simulink model "FTD_test"  (R2023a)
settings: Solver=FixedStepAuto  StartTime=0.0  StopTime=150  FixedStep=0.001  RelTol=1e-3
libraries: simulink x2
settings Model: Creator=邓宇飞  LastModifiedBy=邓宇飞

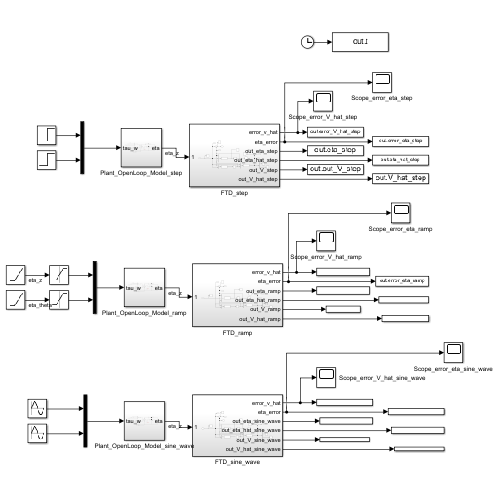
[thumbnail: Simulink's stored preview of the top-level diagram]
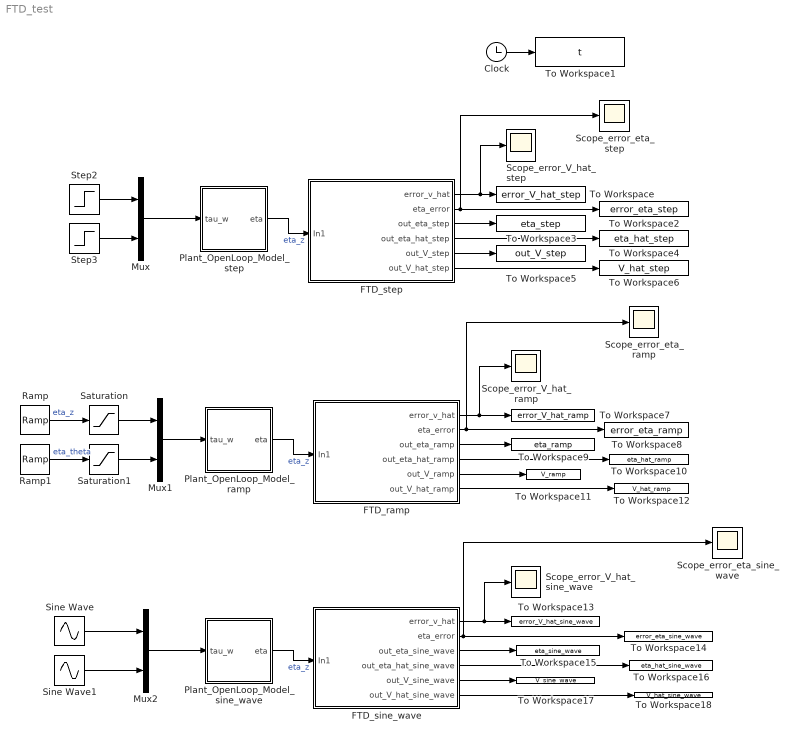
== system FTD_test ==
  Clock : Clock
  FTD_ramp : Subsystem
  FTD_sine_wave : Subsystem
  FTD_step : Subsystem
  Mux : Mux  Inputs=2
  Mux1 : Mux  Inputs=2
  Mux2 : Mux  Inputs=2
  Plant_OpenLoop_Model_ramp : Subsystem
  Plant_OpenLoop_Model_sine_wave : Subsystem
  Plant_OpenLoop_Model_step : Subsystem
  Ramp : simulink/Sources/Ramp  slope=1  start=1  InitialOutput=0
  Ramp1 : simulink/Sources/Ramp  slope=1  start=1  InitialOutput=0
  Saturation : Saturate  UpperLimit=10  LowerLimit=0
  Saturation1 : Saturate  UpperLimit=10  LowerLimit=0
  Scope_error_V_hat_ramp : Scope
  Scope_error_V_hat_sine_wave : Scope
  Scope_error_V_hat_step : Scope
  Scope_error_eta_ramp : Scope
  Scope_error_eta_sine_wave : Scope
  Scope_error_eta_step : Scope
  Sine Wave : Sin  Frequency=0.5*pi  Phase=0.5*pi  SampleTime=0
  Sine Wave1 : Sin  Frequency=0.5*pi  Phase=0.5*pi  SampleTime=0
  Step2 : Step  Time=0  SampleTime=0
  Step3 : Step  Time=0  SampleTime=0
  To Workspace : ToWorkspace  VariableName=error_V_hat_step  SaveFormat=Timeseries  SampleTime=-1
  To Workspace1 : ToWorkspace  VariableName=t  SaveFormat=Timeseries  SampleTime=-1
  To Workspace10 : ToWorkspace  VariableName=eta_hat_ramp  SaveFormat=Timeseries  SampleTime=-1
  To Workspace11 : ToWorkspace  VariableName=V_ramp  SaveFormat=Timeseries  SampleTime=-1
  To Workspace12 : ToWorkspace  VariableName=V_hat_ramp  SaveFormat=Timeseries  SampleTime=-1
  To Workspace13 : ToWorkspace  VariableName=error_V_hat_sine_wave  SaveFormat=Timeseries  SampleTime=-1
  To Workspace14 : ToWorkspace  VariableName=error_eta_sine_wave  SaveFormat=Timeseries  SampleTime=-1
  To Workspace15 : ToWorkspace  VariableName=eta_sine_wave  SaveFormat=Timeseries  SampleTime=-1
  To Workspace16 : ToWorkspace  VariableName=eta_hat_sine_wave  SaveFormat=Timeseries  SampleTime=-1
  To Workspace17 : ToWorkspace  VariableName=V_sine_wave  SaveFormat=Timeseries  SampleTime=-1
  To Workspace18 : ToWorkspace  VariableName=V_hat_sine_wave  SaveFormat=Timeseries  SampleTime=-1
  To Workspace2 : ToWorkspace  VariableName=error_eta_step  SaveFormat=Timeseries  SampleTime=-1
  To Workspace3 : ToWorkspace  VariableName=eta_step  SaveFormat=Timeseries  SampleTime=-1
  To Workspace4 : ToWorkspace  VariableName=eta_hat_step  SaveFormat=Timeseries  SampleTime=-1
  To Workspace5 : ToWorkspace  VariableName=out_V_step  SaveFormat=Timeseries  SampleTime=-1
  To Workspace6 : ToWorkspace  VariableName=V_hat_step  SaveFormat=Timeseries  SampleTime=-1
  To Workspace7 : ToWorkspace  VariableName=error_V_hat_ramp  SaveFormat=Timeseries  SampleTime=-1
  To Workspace8 : ToWorkspace  VariableName=error_eta_ramp  SaveFormat=Timeseries  SampleTime=-1
  To Workspace9 : ToWorkspace  VariableName=eta_ramp  SaveFormat=Timeseries  SampleTime=-1
  wires:
  Plant_OpenLoop_Model_step/1(eta) -> FTD_step/1(In1)  "eta_z"
  FTD_step/1(error_v_hat) -> Scope_error_V_hat_step/1, To Workspace/1
  FTD_step/2(eta_error) -> To Workspace2/1, Scope_error_eta_step/1
  FTD_ramp/2(eta_error) -> To Workspace8/1, Scope_error_eta_ramp/1
  FTD_ramp/1(error_v_hat) -> To Workspace7/1, Scope_error_V_hat_ramp/1
  Plant_OpenLoop_Model_ramp/1(eta) -> FTD_ramp/1(In1)  "eta_z"
  FTD_sine_wave/2(eta_error) -> To Workspace14/1, Scope_error_eta_sine_wave/1
  FTD_sine_wave/1(error_v_hat) -> To Workspace13/1, Scope_error_V_hat_sine_wave/1
  Plant_OpenLoop_Model_sine_wave/1(eta) -> FTD_sine_wave/1(In1)  "eta_z"
  Mux/1 -> Plant_OpenLoop_Model_step/1(tau_w)
  Step2/1 -> Mux/1
  Step3/1 -> Mux/2
  Mux1/1 -> Plant_OpenLoop_Model_ramp/1(tau_w)
  Saturation1/1 -> Mux1/2
  Saturation/1 -> Mux1/1
  Ramp/1 -> Saturation/1  "eta_z"
  Ramp1/1 -> Saturation1/1  "eta_theta"
  Mux2/1 -> Plant_OpenLoop_Model_sine_wave/1(tau_w)
  Sine Wave/1 -> Mux2/1
  Sine Wave1/1 -> Mux2/2
  FTD_step/3(out_eta_step) -> To Workspace3/1
  FTD_step/4(out_eta_hat_step) -> To Workspace4/1
  FTD_step/6(out_V_hat_step) -> To Workspace6/1
  FTD_ramp/3(out_eta_ramp) -> To Workspace9/1
  FTD_ramp/4(out_eta_hat_ramp) -> To Workspace10/1
  FTD_ramp/5(out_V_ramp) -> To Workspace11/1
  FTD_ramp/6(out_V_hat_ramp) -> To Workspace12/1
  FTD_sine_wave/3(out_eta_sine_wave) -> To Workspace15/1
  FTD_sine_wave/4(out_eta_hat_sine_wave) -> To Workspace16/1
  FTD_sine_wave/5(out_V_sine_wave) -> To Workspace17/1
  FTD_sine_wave/6(out_V_hat_sine_wave) -> To Workspace18/1
  Clock/1 -> To Workspace1/1
  FTD_step/5(out_V_step) -> To Workspace5/1

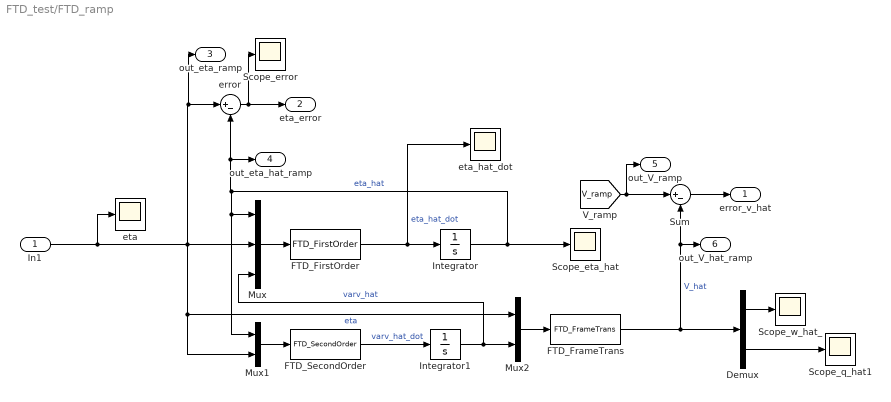
== system FTD_test/FTD_ramp ==
  In1 : Inport
  Demux : Demux  Outputs=2
  FTD_FirstOrder : MATLABFcn  MATLABFcn=FTD_FirstOrder  OutputDimensions=2  OutputSignalType=real
  FTD_FrameTrans : MATLABFcn  MATLABFcn=FTD_FrameTrans  OutputDimensions=2  OutputSignalType=real
  FTD_SecondOrder : MATLABFcn  MATLABFcn=FTD_SecondOrder  OutputDimensions=2  OutputSignalType=real
  Integrator : Integrator
  Integrator1 : Integrator
  Mux : Mux  Inputs=3
  Mux1 : Mux  Inputs=2
  Mux2 : Mux  Inputs=2
  Scope_error : Scope
  Scope_eta_hat : Scope
  Scope_q_hat1 : Scope
  Scope_w_hat_ : Scope
  Sum : Sum  Inputs=|+-
  error : Sum  Inputs=|+-
  eta : Scope
  eta_hat_dot : Scope
  error_v_hat : Outport
  eta_error : Outport  Port=2
  out_eta_ramp : Outport  Port=3
  out_eta_hat_ramp : Outport  Port=4
  out_V_ramp : Outport  Port=5
  out_V_hat_ramp : Outport  Port=6
  wires:
  In1/1 -> eta/1, out_eta_ramp/1, error/1, Mux2/1, Mux1/2, Mux/2  "eta"
  Mux/1 -> FTD_FirstOrder/1
  Integrator/1 -> Scope_eta_hat/1, out_eta_hat_ramp/1, error/2, Mux1/1, Mux/1  "eta_hat"
  FTD_FrameTrans/1 -> Demux/1, out_V_hat_ramp/1, Sum/2  "V_hat"
  FTD_FirstOrder/1 -> Integrator/1, eta_hat_dot/1  "eta_hat_dot"
  error/1 -> eta_error/1, Scope_error/1
  Demux/1 -> Scope_w_hat_/1
  FTD_SecondOrder/1 -> Integrator1/1  "varv_hat_dot"
  Integrator1/1 -> Mux/3, Mux2/2  "varv_hat"
  Mux1/1 -> FTD_SecondOrder/1
  Mux2/1 -> FTD_FrameTrans/1
  Demux/2 -> Scope_q_hat1/1
  [V_ramp] -> out_V_ramp/1, Sum/1
  Sum/1 -> error_v_hat/1

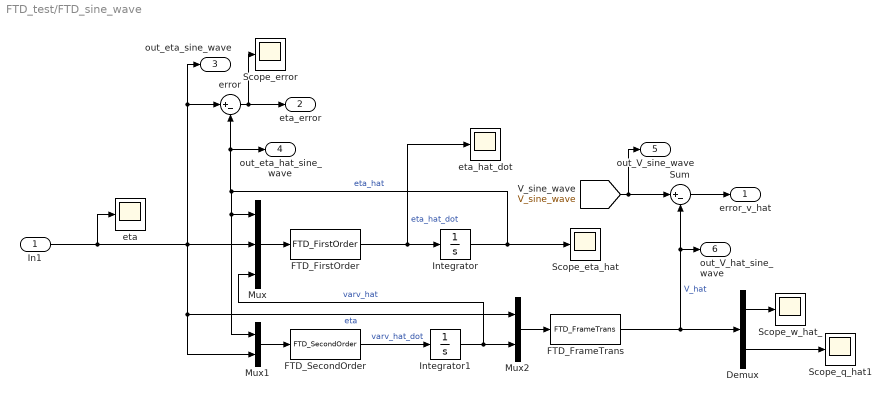
== system FTD_test/FTD_sine_wave ==
  In1 : Inport
  Demux : Demux  Outputs=2
  FTD_FirstOrder : MATLABFcn  MATLABFcn=FTD_FirstOrder  OutputDimensions=2  OutputSignalType=real
  FTD_FrameTrans : MATLABFcn  MATLABFcn=FTD_FrameTrans  OutputDimensions=2  OutputSignalType=real
  FTD_SecondOrder : MATLABFcn  MATLABFcn=FTD_SecondOrder  OutputDimensions=2  OutputSignalType=real
  Integrator : Integrator
  Integrator1 : Integrator
  Mux : Mux  Inputs=3
  Mux1 : Mux  Inputs=2
  Mux2 : Mux  Inputs=2
  Scope_error : Scope
  Scope_eta_hat : Scope
  Scope_q_hat1 : Scope
  Scope_w_hat_ : Scope
  Sum : Sum  Inputs=|+-
  error : Sum  Inputs=|+-
  eta : Scope
  eta_hat_dot : Scope
  error_v_hat : Outport
  eta_error : Outport  Port=2
  out_eta_sine_wave : Outport  Port=3
  out_eta_hat_sine_wave : Outport  Port=4
  out_V_sine_wave : Outport  Port=5
  out_V_hat_sine_wave : Outport  Port=6
  wires:
  In1/1 -> eta/1, out_eta_sine_wave/1, error/1, Mux2/1, Mux1/2, Mux/2  "eta"
  Mux/1 -> FTD_FirstOrder/1
  Integrator/1 -> Scope_eta_hat/1, out_eta_hat_sine_wave/1, error/2, Mux1/1, Mux/1  "eta_hat"
  FTD_FrameTrans/1 -> Demux/1, out_V_hat_sine_wave/1, Sum/2  "V_hat"
  FTD_FirstOrder/1 -> Integrator/1, eta_hat_dot/1  "eta_hat_dot"
  error/1 -> eta_error/1, Scope_error/1
  Demux/1 -> Scope_w_hat_/1
  FTD_SecondOrder/1 -> Integrator1/1  "varv_hat_dot"
  Integrator1/1 -> Mux/3, Mux2/2  "varv_hat"
  Mux1/1 -> FTD_SecondOrder/1
  Mux2/1 -> FTD_FrameTrans/1
  Demux/2 -> Scope_q_hat1/1
  [V_sine_wave] -> out_V_sine_wave/1, Sum/1
  Sum/1 -> error_v_hat/1

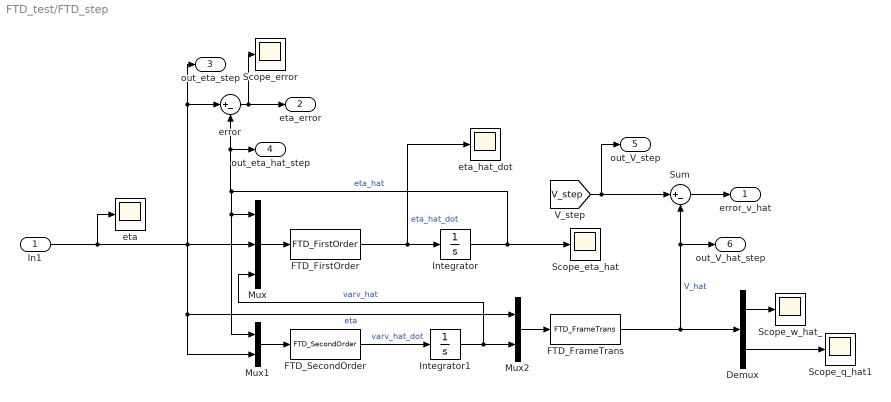
== system FTD_test/FTD_step ==
  In1 : Inport
  Demux : Demux  Outputs=2
  FTD_FirstOrder : MATLABFcn  MATLABFcn=FTD_FirstOrder  OutputDimensions=2  OutputSignalType=real
  FTD_FrameTrans : MATLABFcn  MATLABFcn=FTD_FrameTrans  OutputDimensions=2  OutputSignalType=real
  FTD_SecondOrder : MATLABFcn  MATLABFcn=FTD_SecondOrder  OutputDimensions=2  OutputSignalType=real
  Integrator : Integrator
  Integrator1 : Integrator
  Mux : Mux  Inputs=3
  Mux1 : Mux  Inputs=2
  Mux2 : Mux  Inputs=2
  Scope_error : Scope
  Scope_eta_hat : Scope
  Scope_q_hat1 : Scope
  Scope_w_hat_ : Scope
  Sum : Sum  Inputs=|+-
  error : Sum  Inputs=|+-
  eta : Scope
  eta_hat_dot : Scope
  error_v_hat : Outport
  eta_error : Outport  Port=2
  out_eta_step : Outport  Port=3
  out_eta_hat_step : Outport  Port=4
  out_V_step : Outport  Port=5
  out_V_hat_step : Outport  Port=6
  wires:
  In1/1 -> eta/1, error/1, out_eta_step/1, Mux2/1, Mux1/2, Mux/2  "eta"
  Mux/1 -> FTD_FirstOrder/1
  Integrator/1 -> Scope_eta_hat/1, out_eta_hat_step/1, error/2, Mux1/1, Mux/1  "eta_hat"
  FTD_FrameTrans/1 -> Demux/1, out_V_hat_step/1, Sum/2  "V_hat"
  FTD_FirstOrder/1 -> Integrator/1, eta_hat_dot/1  "eta_hat_dot"
  error/1 -> eta_error/1, Scope_error/1
  Demux/1 -> Scope_w_hat_/1
  FTD_SecondOrder/1 -> Integrator1/1  "varv_hat_dot"
  Integrator1/1 -> Mux/3, Mux2/2  "varv_hat"
  Mux1/1 -> FTD_SecondOrder/1
  Mux2/1 -> FTD_FrameTrans/1
  Demux/2 -> Scope_q_hat1/1
  [V_step] -> Sum/1, out_V_step/1
  Sum/1 -> error_v_hat/1

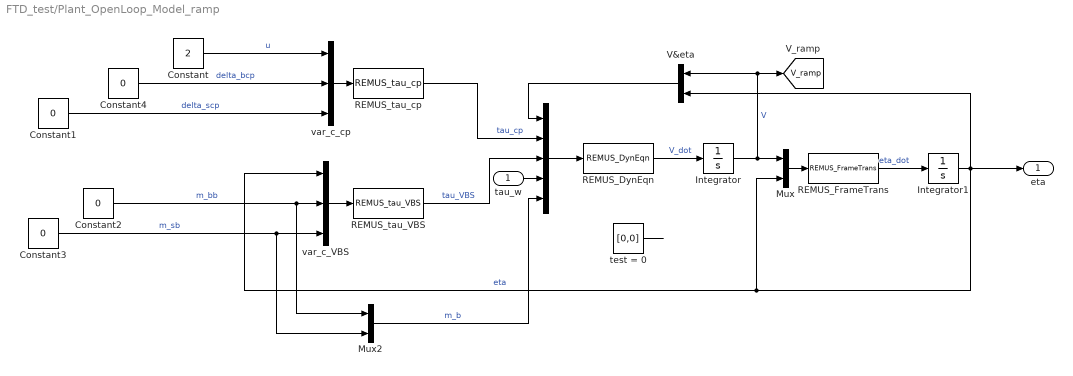
== system FTD_test/Plant_OpenLoop_Model_ramp ==
  tau_w : Inport
  " " : Mux  Inputs=5
  Constant : Constant  Value=2  OutDataTypeStr=Inherit: Inherit via back propagation
  Constant{1..4} (4 alike) : Constant  Value=0
  Integrator : Integrator
  Integrator1 : Integrator
  Mux : Mux  Inputs=2
  Mux2 : Mux  Inputs=2
  REMUS_DynEqn : MATLABFcn  MATLABFcn=REMUS_DynEqn  OutputDimensions=2  OutputSignalType=real
  REMUS_FrameTrans : MATLABFcn  MATLABFcn=REMUS_FrameTrans  OutputDimensions=2  OutputSignalType=real
  REMUS_tau_VBS : MATLABFcn  MATLABFcn=REMUS_tau_VBS  OutputDimensions=2  OutputSignalType=real
  REMUS_tau_cp : MATLABFcn  MATLABFcn=REMUS_tau_cp  OutputDimensions=2  OutputSignalType=real
  V&eta : Mux  Inputs=2
  test = 0 : Constant  Value=[0,0]
  var_c_VBS : Mux  Inputs=3
  var_c_cp : Mux  Inputs=3
  eta : Outport
  tag scope: V_ramp=global
  wires:
  Constant/1 -> var_c_cp/1  "u"
  REMUS_DynEqn/1 -> Integrator/1  "V_dot"
  REMUS_tau_cp/1 -> " "/2  "tau_cp"
  Integrator1/1 -> eta/1, Mux/2, var_c_VBS/1, V&eta/2  "eta"
  Constant1/1 -> var_c_cp/3  "delta_scp"
  test = 0/1 -> ?
  Constant3/1 -> Mux2/2, var_c_VBS/3  "m_sb"
  Mux/1 -> REMUS_FrameTrans/1
  " "/1 -> REMUS_DynEqn/1
  Integrator/1 -> Mux/1, V&eta/1, [V_ramp]  "V"
  Constant2/1 -> Mux2/1, var_c_VBS/2  "m_bb"
  Constant4/1 -> var_c_cp/2  "delta_bcp"
  var_c_cp/1 -> REMUS_tau_cp/1
  V&eta/1 -> " "/1
  REMUS_tau_VBS/1 -> " "/3  "tau_VBS"
  tau_w/1 -> " "/4
  REMUS_FrameTrans/1 -> Integrator1/1  "eta_dot"
  var_c_VBS/1 -> REMUS_tau_VBS/1
  Mux2/1 -> " "/5  "m_b"

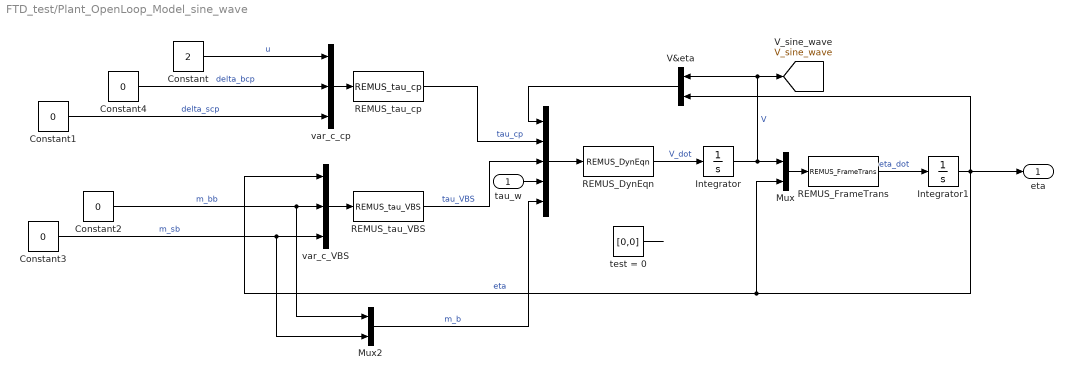
== system FTD_test/Plant_OpenLoop_Model_sine_wave ==
  tau_w : Inport
  " " : Mux  Inputs=5
  Constant : Constant  Value=2  OutDataTypeStr=Inherit: Inherit via back propagation
  Constant{1..4} (4 alike) : Constant  Value=0
  Integrator : Integrator
  Integrator1 : Integrator
  Mux : Mux  Inputs=2
  Mux2 : Mux  Inputs=2
  REMUS_DynEqn : MATLABFcn  MATLABFcn=REMUS_DynEqn  OutputDimensions=2  OutputSignalType=real
  REMUS_FrameTrans : MATLABFcn  MATLABFcn=REMUS_FrameTrans  OutputDimensions=2  OutputSignalType=real
  REMUS_tau_VBS : MATLABFcn  MATLABFcn=REMUS_tau_VBS  OutputDimensions=2  OutputSignalType=real
  REMUS_tau_cp : MATLABFcn  MATLABFcn=REMUS_tau_cp  OutputDimensions=2  OutputSignalType=real
  V&eta : Mux  Inputs=2
  test = 0 : Constant  Value=[0,0]
  var_c_VBS : Mux  Inputs=3
  var_c_cp : Mux  Inputs=3
  eta : Outport
  tag scope: V_sine_wave=global
  wires:
  Constant/1 -> var_c_cp/1  "u"
  REMUS_DynEqn/1 -> Integrator/1  "V_dot"
  REMUS_tau_cp/1 -> " "/2  "tau_cp"
  Integrator1/1 -> eta/1, Mux/2, var_c_VBS/1, V&eta/2  "eta"
  Constant1/1 -> var_c_cp/3  "delta_scp"
  test = 0/1 -> ?
  Constant3/1 -> Mux2/2, var_c_VBS/3  "m_sb"
  Mux/1 -> REMUS_FrameTrans/1
  " "/1 -> REMUS_DynEqn/1
  Integrator/1 -> Mux/1, V&eta/1, [V_sine_wave]  "V"
  Constant2/1 -> Mux2/1, var_c_VBS/2  "m_bb"
  Constant4/1 -> var_c_cp/2  "delta_bcp"
  var_c_cp/1 -> REMUS_tau_cp/1
  V&eta/1 -> " "/1
  REMUS_tau_VBS/1 -> " "/3  "tau_VBS"
  tau_w/1 -> " "/4
  REMUS_FrameTrans/1 -> Integrator1/1  "eta_dot"
  var_c_VBS/1 -> REMUS_tau_VBS/1
  Mux2/1 -> " "/5  "m_b"

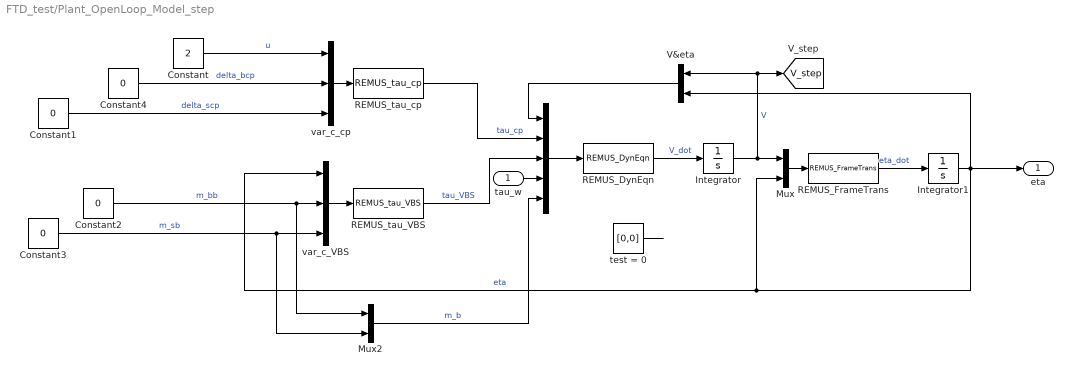
== system FTD_test/Plant_OpenLoop_Model_step ==
  tau_w : Inport
  " " : Mux  Inputs=5
  Constant : Constant  Value=2  OutDataTypeStr=Inherit: Inherit via back propagation
  Constant{1..4} (4 alike) : Constant  Value=0
  Integrator : Integrator
  Integrator1 : Integrator
  Mux : Mux  Inputs=2
  Mux2 : Mux  Inputs=2
  REMUS_DynEqn : MATLABFcn  MATLABFcn=REMUS_DynEqn  OutputDimensions=2  OutputSignalType=real
  REMUS_FrameTrans : MATLABFcn  MATLABFcn=REMUS_FrameTrans  OutputDimensions=2  OutputSignalType=real
  REMUS_tau_VBS : MATLABFcn  MATLABFcn=REMUS_tau_VBS  OutputDimensions=2  OutputSignalType=real
  REMUS_tau_cp : MATLABFcn  MATLABFcn=REMUS_tau_cp  OutputDimensions=2  OutputSignalType=real
  V&eta : Mux  Inputs=2
  test = 0 : Constant  Value=[0,0]
  var_c_VBS : Mux  Inputs=3
  var_c_cp : Mux  Inputs=3
  eta : Outport
  tag scope: V_step=global
  wires:
  Constant/1 -> var_c_cp/1  "u"
  REMUS_DynEqn/1 -> Integrator/1  "V_dot"
  REMUS_tau_cp/1 -> " "/2  "tau_cp"
  Integrator1/1 -> eta/1, Mux/2, var_c_VBS/1, V&eta/2  "eta"
  Constant1/1 -> var_c_cp/3  "delta_scp"
  test = 0/1 -> ?
  Constant3/1 -> Mux2/2, var_c_VBS/3  "m_sb"
  Mux/1 -> REMUS_FrameTrans/1
  " "/1 -> REMUS_DynEqn/1
  Integrator/1 -> Mux/1, V&eta/1, [V_step]  "V"
  Constant2/1 -> Mux2/1, var_c_VBS/2  "m_bb"
  Constant4/1 -> var_c_cp/2  "delta_bcp"
  var_c_cp/1 -> REMUS_tau_cp/1
  V&eta/1 -> " "/1
  REMUS_tau_VBS/1 -> " "/3  "tau_VBS"
  tau_w/1 -> " "/4
  REMUS_FrameTrans/1 -> Integrator1/1  "eta_dot"
  var_c_VBS/1 -> REMUS_tau_VBS/1
  Mux2/1 -> " "/5  "m_b"
